simulink model "wavenew"  (R2024b)
settings: Solver=VariableStepAuto  StartTime=0.0  StopTime=60  RelTol=1e-3
settings Model: Creator=lenovo  LastModifiedBy=lenovo

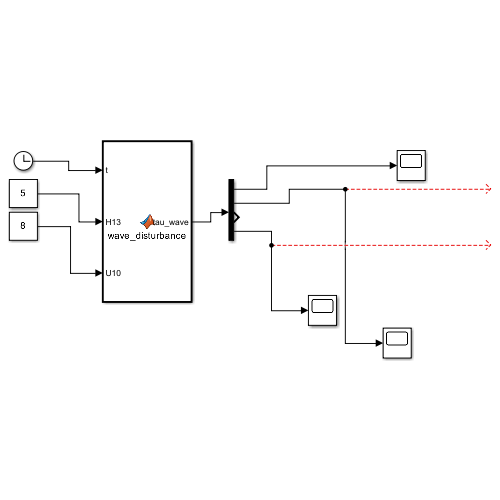
[thumbnail: Simulink's stored preview of the top-level diagram]
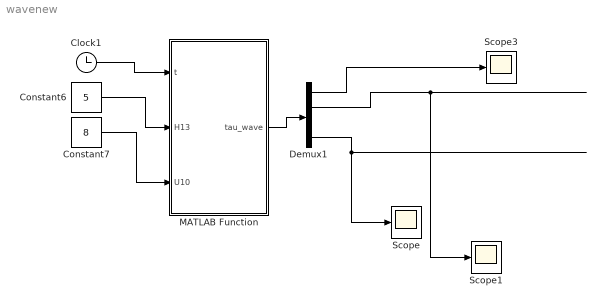
== system wavenew ==
  Clock1 : Clock
  Constant6 : Constant  Value=5
  Constant7 : Constant  Value=8
  Demux1 : Demux
  MATLAB Function : MATLAB Function  TreatAsAtomicUnit=on
  Scope : Scope
  Scope1 : Scope
  Scope3 : Scope
  wires:
  Constant6/1 -> MATLAB Function/2(H13)
  Clock1/1 -> MATLAB Function/1(t)
  Constant7/1 -> MATLAB Function/3(U10)
  MATLAB Function/1(tau_wave) -> Demux1/1
  Demux1/1 -> Scope3/1
  Demux1/2 -> Scope1/1
  Demux1/4 -> Scope/1

== matlab function wavenew/MATLAB Function ==
  data: t input; tau_wave output; H13 input; U10 input
function tau_wave = wave_disturbance(t, H13, U10)
    % 计算波浪干扰力矩
    % 输入参数：
    % t         - 时间 [s]
    % H13       - 有效波高 [m]
    % U10       - 风速 [m/s]
    % beta      - 船舶与海浪的遭遇角 [rad]
    
    % 常数定义
    g = 9.81;               % 重力加速度, m/s^2
    alpha_pm = 8.11e-3;     % Pierson-Moskowitz谱参数
    beta_pm = 3.11;         % Pierson-Moskowitz谱参数
    beta=pi/3;
    % 计算峰值频率
    omega_peak = 0.84 * (g / U10)^(1/3); % 峰值频率, rad/s
    
    % 根据H13确定频率范围和步长
    if H13 <= 2.5
        omegab = 0.3;
        omegal = 3.0;
        delta_omega = 0.1;
    elseif H13 <= 5.0
        omegab = 0.25;
        omegal = 2.4;
        delta_omega = 0.08;
    else 
        omegab = 0.1;
        omegal = 1.7;
        delta_omega = 0.06;
    end
    omega = omegab:delta_omega:omegal;
    
    % 计算海浪能谱
    S_omega = alpha_pm * g^2 ./ omega.^5 .* exp(-beta_pm ./ (H13^2 * omega.^4));
    
    % 计算各频率成分的振幅和相位
    A = sqrt(2 * S_omega * delta_omega);
    phi = rand(1, length(omega)) * 2 * pi; % 随机相位
    
    % 船舶参数
    rho = 1024; % 海水密度 [kg/m^3]
    L = 3.5;     % 船长 [m]
    B = 0.8;     % 船宽 [m]
    D = 0.4;     % 吃水深度 [m]
    
    % 初始化波浪干扰力矩分量
    tao1 = zeros(size(t));
    tao2 = zeros(size(t));
    tao3 = zeros(size(t)); % 第三分量保持为零
    tao4 = zeros(size(t));
    
    % 计算各频率成分对力矩的贡献
    for i = 1:length(omega)
        k = omega(i)^2 / g;           % 波数（深水条件）
        omega_e = omega(i);           % 遭遇频率（假设船速为零）
        phase = omega_e * t + phi(i); % 相位项
        slope_term = k * A(i) * sin(phase); % 波面斜率相关项
        
        % 纵向力矩
        tao1 = tao1 + rho * g * B * L * D * cos(beta) * slope_term;
        % 横向力矩
        tao2 = tao2 - rho * g * B * L * D * sin(beta) * slope_term;
        % 横摇力矩（假设公式正确性）
        tao4 = tao4 + (1/24) * rho * g * B * L * (L^2 - B^2) * sin(2*beta) * (slope_term)^2;
    end
    
    % 组合力矩分量
    tau_wave = [tao1; tao2; tao3; tao4];
end
